simulink model "Constanttobits"  (R2014a)
settings: Solver=ode45  StartTime=0.0  StopTime=10.0  RelTol=1e-3
libraries: hdlsllib x8
settings Model: Creator=Andrew  LastModifiedBy=Andrew

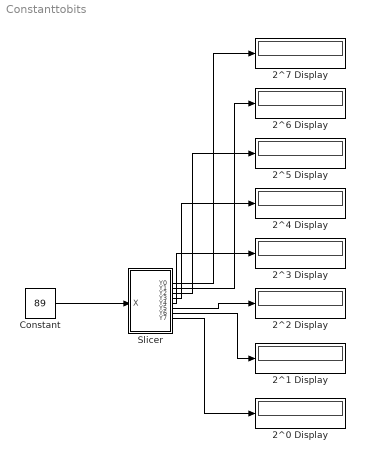
== system Constanttobits ==
  2^0 Display : Display
  2^1 Display : Display
  2^2 Display : Display
  2^3 Display : Display
  2^4 Display : Display
  2^5 Display : Display
  2^6 Display : Display
  2^7 Display : Display
  Constant : Constant  Value=89  OutDataTypeStr=int8
  Slicer : Subsystem
  wires:
  Constant/1 -> Slicer/1(X)
  Slicer/1(Y0) -> 2^7 Display/1
  Slicer/2(Y1) -> 2^6 Display/1
  Slicer/3(Y2) -> 2^5 Display/1
  Slicer/4(Y3) -> 2^4 Display/1
  Slicer/5(Y4) -> 2^3 Display/1
  Slicer/6(Y5) -> 2^2 Display/1
  Slicer/7(Y6) -> 2^1 Display/1
  Slicer/8(Y7) -> 2^0 Display/1

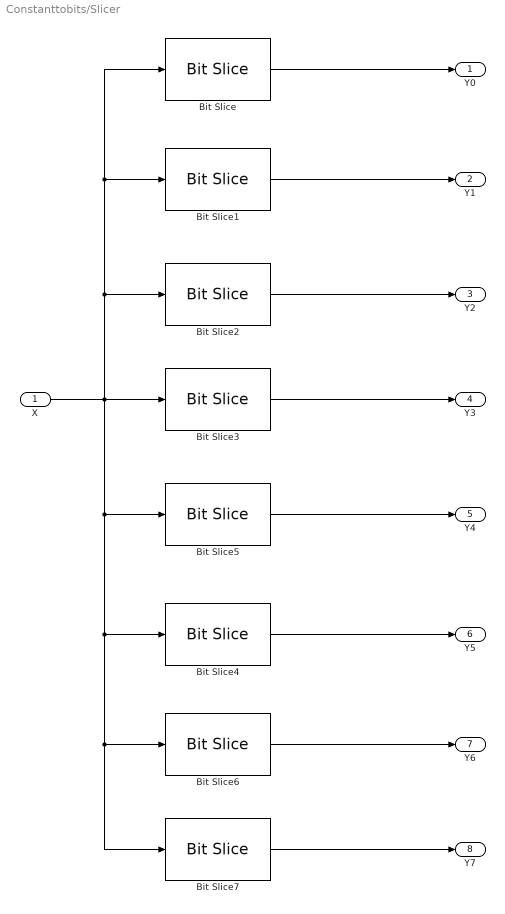
== system Constanttobits/Slicer ==
  X : Inport  OutDataTypeStr=int8  SampleTime=1
  Bit Slice : hdlsllib/HDL Operations/Bit Slice  lidx=7  ridx=7
  Bit Slice1 : hdlsllib/HDL Operations/Bit Slice  lidx=6  ridx=6
  Bit Slice2 : hdlsllib/HDL Operations/Bit Slice  lidx=5  ridx=5
  Bit Slice3 : hdlsllib/HDL Operations/Bit Slice  lidx=4  ridx=4
  Bit Slice4 : hdlsllib/HDL Operations/Bit Slice  lidx=2  ridx=2
  Bit Slice5 : hdlsllib/HDL Operations/Bit Slice  lidx=3  ridx=3
  Bit Slice6 : hdlsllib/HDL Operations/Bit Slice  lidx=1  ridx=1
  Bit Slice7 : hdlsllib/HDL Operations/Bit Slice  lidx=0  ridx=0
  Y0 : Outport
  Y1 : Outport  Port=2
  Y2 : Outport  Port=3
  Y3 : Outport  Port=4
  Y4 : Outport  Port=5
  Y5 : Outport  Port=6
  Y6 : Outport  Port=7
  Y7 : Outport  Port=8
  wires:
  X/1 -> Bit Slice7/1, Bit Slice6/1, Bit Slice4/1, Bit Slice5/1, Bit Slice/1, Bit Slice1/1, Bit Slice2/1, Bit Slice3/1
  Bit Slice/1 -> Y0/1
  Bit Slice7/1 -> Y7/1
  Bit Slice3/1 -> Y3/1
  Bit Slice1/1 -> Y1/1
  Bit Slice5/1 -> Y4/1
  Bit Slice2/1 -> Y2/1
  Bit Slice4/1 -> Y5/1
  Bit Slice6/1 -> Y6/1
